simulink model "L0205"  (R2015b)
settings: Solver=VariableStepAuto  StartTime=0.0  StopTime=10.0  RelTol=1e-3
libraries: simulink x4
settings Model: Creator=mmf.shpakAV  LastModifiedBy=mmf.shpakAV

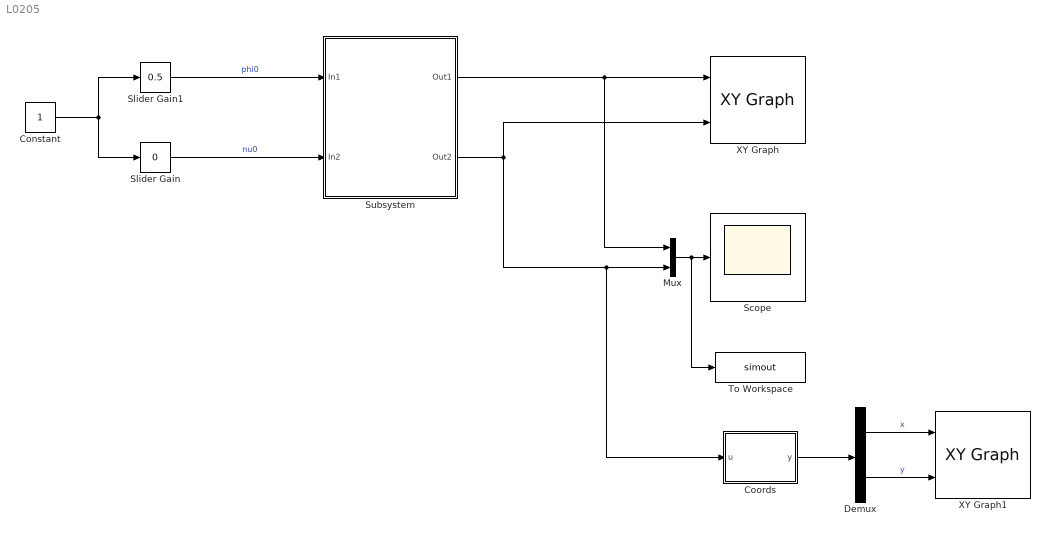
== system L0205 ==
  Constant : Constant
  Coords : MATLAB Function  TreatAsAtomicUnit=on
  Demux : Demux  Outputs=2
  Mux : Mux  Inputs=2
  Scope : Scope
  Slider Gain : simulink/Math Operations/Slider Gain  low=0  gain=0  high=2
  Slider Gain1 : simulink/Math Operations/Slider Gain  low=0  gain=0.5  high=2
  Subsystem : Subsystem
  To Workspace : ToWorkspace  VariableName=simout  SaveFormat=Structure With Time  SampleTime=-1
  XY Graph : simulink/Sinks/XY Graph  xmin=-1  xmax=1  ymin=-1  ymax=1  st=-1
  XY Graph1 : simulink/Sinks/XY Graph  xmin=-1  xmax=1  ymin=-1  ymax=1  st=-1
  wires:
  Mux/1 -> To Workspace/1, Scope/1
  Demux/1 -> XY Graph1/1  "x"
  Demux/2 -> XY Graph1/2  "y"
  Coords/1(y) -> Demux/1
  Constant/1 -> Slider Gain/1, Slider Gain1/1
  Subsystem/2(Out2) -> XY Graph/2, Coords/1(u), Mux/2
  Subsystem/1(Out1) -> Mux/1, XY Graph/1
  Slider Gain1/1 -> Subsystem/1(In1)  "phi0"
  Slider Gain/1 -> Subsystem/2(In2)  "nu0"

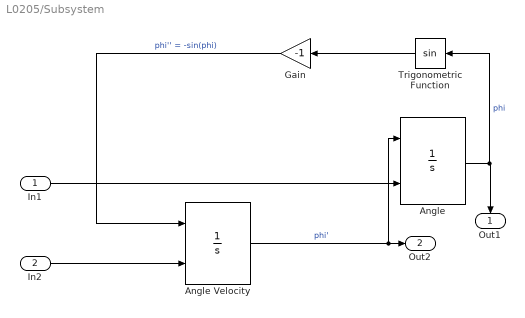
== system L0205/Subsystem ==
  In1 : Inport
  In2 : Inport  Port=2
  Angle : Integrator  InitialConditionSource=external
  Angle Velocity : Integrator  InitialConditionSource=external
  Gain : Gain  Gain=-1
  Trigonometric Function : Trigonometry
  Out1 : Outport
  Out2 : Outport  Port=2
  wires:
  Angle Velocity/1 -> Angle/1, Out2/1  "phi'"
  Angle/1 -> Out1/1, Trigonometric Function/1  "phi"
  Gain/1 -> Angle Velocity/1  "phi'' = -sin(phi)"
  In2/1 -> Angle Velocity/2
  In1/1 -> Angle/2
  Trigonometric Function/1 -> Gain/1

== matlab function L0205/Coords ==
  data: u input; y output
function y  = fcn(u)
%#codegen

y = [cos(u),-sin(u)]';
